simulink model "adaptive_mpc_controller"  (R2023b)
settings: Solver=VariableStepAuto  StartTime=0.0  StopTime=15  FixedStep=0.01  RelTol=1e-3
libraries: mpclib x1, Meldas_library x1
settings Model: Creator=mulusoy  LastModifiedBy=omp31
settings SolverCC: AlgebraicLoopSolver=TrustRegion
settings DataIOCC: ReturnWorkspaceOutputs=off
settings OptimizationCC: DefaultParameterBehavior=Inlined  EnhancedBackFolding=on  PassReuseOutputArgsAs=Individual arguments  OptimizeBlockOrder=speed  DifferentSizesBufferReuse=on  OptimizationCustomize=off  EfficientTunableParamExpr=on
settings DebuggingCC: ParameterTunabilityLossMsg=error  UnconnectedInputMsg=warning  UnconnectedOutputMsg=warning  UnconnectedLineMsg=warning  ArithmeticOperatorsInVariantConditions=warning
settings ModelReferenceCC: EnableRefExpFcnMdlSchedulingChecks=on
settings SFSimCC: SimUseLocalCustomCode=off  MATLABDynamicMemAlloc=off  CustomCodeUndefinedFunction=UseInterfaceOnly
settings RTWCC: Description=Embedded Coder  SystemTargetFile=ert.tlc  TemplateMakefile=ert_default_tmf  GenerateReport=on  RTWUseLocalCustomCode=off  IncludeHyperlinkInReport=on  LaunchReport=on  GenerateTraceInfo=on  GenerateTraceReport=on  GenerateTraceReportSl=on  GenerateTraceReportSf=on  GenerateTraceReportEml=on
settings CodeAppCC: ForceParamTrailComments=on  IgnoreCustomStorageClasses=off  OperatorAnnotations=on  SimulinkDataObjDesc=on  SFDataObjDesc=on  InsertBlockDesc=on
settings ERTTargetCC: TargetLangStandard=C99 (ISO)  GenerateSampleERTMain=on  InlinedParameterPlacement=NonHierarchical  ERTCustomFileTemplate=example_file_process.tlc

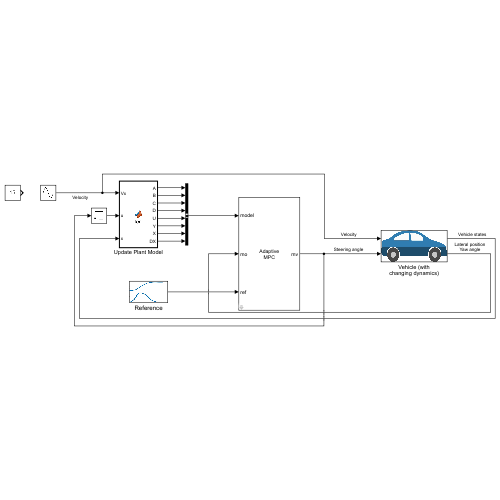
[thumbnail: Simulink's stored preview of the top-level diagram]
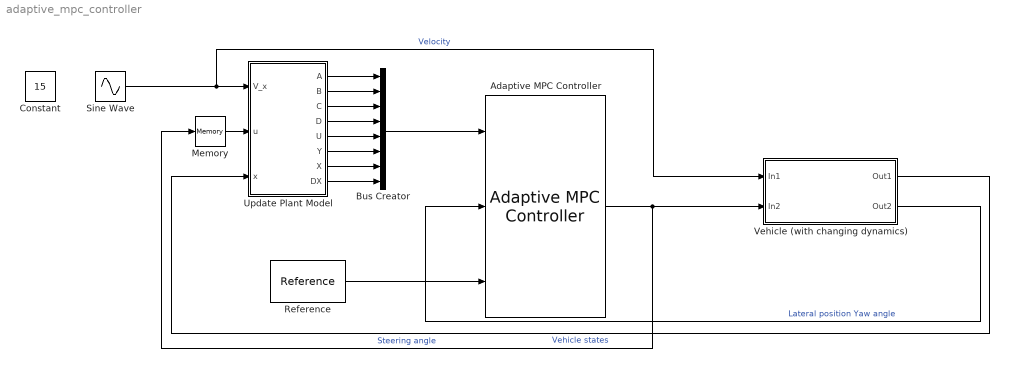
== system adaptive_mpc_controller ==
  Adaptive MPC Controller : mpclib/Adaptive MPC Controller  SCDEnableBlockLinearizationSpecification=on  mpcobj=mpc1  enable_value=0  updateMPCinCallerWorkspace=on  md_inport=off  mv_inport=off  uref_inport=off  return_cost=off  return_mvseq=off  return_qpstatus=off  return_xseq=off  return_state=off  return_ovseq=off  state_inport=off  isltv_plant=off  umin_inport=off  umax_inport=off  ymin_inport=off  ymax_inport=off  cc_inport=off  ywt_inport=off  uwt_inport=off  duwt_inport=off  rhoeps_inport=off  pm_inport=off  MaximumP=10  HorizonChoice=FixedHorizon  BlockDataType=double  SampleTimeInherited=off  switch_inport=off
  Bus Creator : BusCreator  Inputs=8
  Constant : Constant  Value=15
  Memory : Memory
  Reference : Meldas_library/Reference  SystemSampleTime=-1  VariantActivationTime=update diagram  AllowFlexibleInterface=on  Latency=0  AutoFrameSizeCalculation=off
  Sine Wave : Sin  Amplitude=20  Bias=5  Frequency=0.2  SampleTime=0
  Update Plant Model : MATLAB Function  TreatAsAtomicUnit=on
  Vehicle (with changing dynamics) : Subsystem
      mask Display: image('car.jpg');
  wires:
  Sine Wave/1 -> Vehicle (with changing dynamics)/1(In1), Update Plant Model/1(V_x)  "Velocity"
  Update Plant Model/1(A) -> Bus Creator/1
  Update Plant Model/2(B) -> Bus Creator/2
  Update Plant Model/3(C) -> Bus Creator/3
  Update Plant Model/4(D) -> Bus Creator/4
  Update Plant Model/5(U) -> Bus Creator/5
  Update Plant Model/6(Y) -> Bus Creator/6
  Update Plant Model/7(X) -> Bus Creator/7
  Update Plant Model/8(DX) -> Bus Creator/8
  Bus Creator/1 -> Adaptive MPC Controller/1
  Adaptive MPC Controller/1 -> Memory/1, Vehicle (with changing dynamics)/2(In2)  "Steering angle"
  Reference/1 -> Adaptive MPC Controller/3
  Vehicle (with changing dynamics)/2(Out2) -> Adaptive MPC Controller/2  "Lateral position Yaw angle"
  Vehicle (with changing dynamics)/1(Out1) -> Update Plant Model/3(x)  "Vehicle states"
  Memory/1 -> Update Plant Model/2(u)

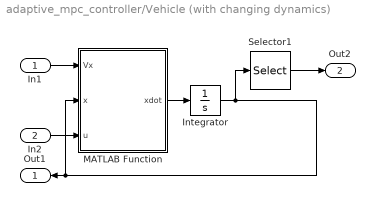
== system adaptive_mpc_controller/Vehicle (with changing dynamics) ==
  In1 : Inport
  In2 : Inport  Port=2
  Integrator : Integrator
  MATLAB Function : MATLAB Function  TreatAsAtomicUnit=on
  Selector1 : Selector  InputPortWidth=4  IndexOptions=Index vector (dialog)  Indices=[4 2]  OutputSizes=1
  Out1 : Outport  VectorParamsAs1DForOutWhenUnconnected=off
  Out2 : Outport  Port=2  VectorParamsAs1DForOutWhenUnconnected=off
  wires:
  In2/1 -> MATLAB Function/3(u)
  In1/1 -> MATLAB Function/1(Vx)
  Integrator/1 -> Selector1/1, MATLAB Function/2(x), Out1/1
  MATLAB Function/1(xdot) -> Integrator/1
  Selector1/1 -> Out2/1

== matlab function adaptive_mpc_controller/Vehicle (with changing dynamics)/MATLAB Function ==
  data: Vx input; x input size=[4,1]; u input; xdot output size=[4,1]
function xdot = fcn(Vx,x,u)

% Model parameters
m = 1575;
Iz = 2875;
lf = 1.2;
lr = 1.6;
Cf = 19000;
Cr = 33000;

% Continuous-time model
A = [-(2*Cf+2*Cr)/m/Vx, 0, -Vx-(2*Cf*lf-2*Cr*lr)/m/Vx, 0;
     0, 0, 1, 0;
     -(2*Cf*lf-2*Cr*lr)/Iz/Vx, 0, -(2*Cf*lf^2+2*Cr*lr^2)/Iz/Vx, 0;
     1, Vx, 0, 0];
B = [2*Cf/m 0 2*Cf*lf/Iz 0]';   
C = [0 0 0 1; 0 1 0 0];
D = zeros(2,1);
xdot = A*x + B*u;
%y = C*x + D*u;

== matlab function adaptive_mpc_controller/Update Plant Model ==
  data: V_x input; u input; A output size=[4,4]; x input size=[4,1]; B output size=[4,1]; C output size=[2,4]; D output size=[2,1]; U output; Y output size=[2,1]; X output size=[4,1]; DX output size=[4,1]
function [A, B, C, D, U, Y, X, DX] = tf_fn(V_x, u, x)
% define the vehicle parameters
m = 1600;
I_z = 2750;
C_f = 19000;
l_f = 1.2;
C_r = 33000;
l_r = 1.6;

% define the controller sample time
Ts = 0.1;

% vehicle dynamics equations to compute a continuous-time model
A_c = [-2*(C_f+C_r) / (V_x*m), 0, -V_x - (2*(C_f*lf-C_r*l_r)) / (V_x*m), 0;
     0, 0, 1, 0;
     -2*(C_f*lf-C_r*l_r) / (V_x*Iz), 0, -2*(C_f*lf^2+C_r*l_r^2) / (V_x*Iz), 0;
     1, V_x, 0, 0];
B_c = [2*C_f/m 0 2*C_f*lf/Iz 0]';   
C_c = [0 0 0 1; 0 1 0 0];
D_c = zeros(2,1);

% generate discrete-time model from the CT model
nx = size(Ac,1);
nu = size(Bc,2);

% compute the matrix exponential using the eigenvalues of the corresponding
% state matrices
M = expm([[A_c B_c]*Ts; zeros(nu, nx+nu)]);
A = M(1:nx, 1:nx);
B = M(1:nx, nx+1:nx+nu);
C = C_c;
D = D_c;

% updated states for the discrete-time plant
X = x;
U = u;
Y = C*x + D*u;
DX = A*x + B*u - x;
